simulink model "QuarterCarSuspension_JAM"  (R2024b)
settings: Solver=ode45  StartTime=0.0  StopTime=10  MaxStep=0.01  RelTol=1e-3  AbsTol=1e-6
StopFcn:
  | if exist('sldemo_suspn_output')
  | sldemo_suspgraph
  | end
model workspace (MATLAB code in the model file):
  | sldemo_suspdat; %load data from file
values from neighbouring files (symbols this model uses):
  cs = 2500    [QuarterCar_dat.m]
  ks = 28000    [QuarterCar_dat.m]
  kt = 190000    [QuarterCar_dat.m]
  Mb = 300    [QuarterCar_dat.m]
  Mu = 40    [QuarterCar_dat.m]
CloseFcn:
  | if exist('suspnFigH')
  |   if ishghandle(suspnFigH,'figure')
  |     close(suspnFigH)
  |   end
  |   clear suspnFigH
  | end
  | if exist('suspnAxH'), clear suspnAxH; end
Description:
  | Automotive Suspension
  | 
  | This example shows how to model a simplified half-car model that includes an independent
  | front and rear vertical suspension. The model also includes body pitch and
  | bounce degrees of freedom. The example provides a description of the model to
  | show how simulation can be used for investigating ride characteristics.
  | In conjunction with a powertrain simulation, the model could
  | investigate longitudinal shuffle resulting from changes in throttle setting.
settings Model: ModifiedByFormat=The MathWorks, Inc.  Creator=The MathWorks, Inc.  LastModifiedBy=The MathWorks, Inc.
settings SolverCC: AutoScaleAbsTol=off  AlgebraicLoopSolver=TrustRegion  MaxZcPerStep=1
settings DataIOCC: InitialState=x0  SaveFormat=StructureWithTime  SaveOutput=off  SaveTime=off  ReturnWorkspaceOutputs=off  StateSaveName=x  TimeSaveName=t  SignalLoggingName=sldemo_suspn_output
settings OptimizationCC: ReuseModelBlockBuffer=off  ExpressionDepthLimit=2147483647  InitFltsAndDblsToZero=on  LifeSpan=inf  BufferReusableBoundary=off
settings DebuggingCC: SaveWithParameterizedLinksMsg=none  SignalResolutionControl=TryResolveAllWithWarning  MultiTaskDSMMsg=warning  SigSpecEnsureSampleTimeMsg=none  IntegerOverflowMsg=none  FcnCallInpInsideContextMsg=warning  UnconnectedInputMsg=warning  UnconnectedOutputMsg=warning  UnconnectedLineMsg=warning  BusObjectLabelMismatch=none  StateNameClashWarn=warning  SFUnexpectedBacktrackingDiag=warning  SFNoUnconditionalDefaultTransitionDiag=warning  SFExecutionAtInitializationDiag=none  IntegerSaturationMsg=none  ArithmeticOperatorsInVariantConditions=warning
settings HardwareCC: ProdBitPerPointer=32  ProdBitPerSizeT=32  ProdBitPerPtrDiffT=32  ProdLargestAtomicFloat=None  ProdIntDivRoundTo=Undefined  ProdEndianess=Unspecified  ProdWordSize=32  ProdHWDeviceType=32-bit Generic
settings ModelReferenceCC: EnableRefExpFcnMdlSchedulingChecks=on  PropagateSignalLabelsOutOfModel=off
settings SFSimCC: SimUseLocalCustomCode=off  CustomCodeUndefinedFunction=UseInterfaceOnly
settings RTWCC: RTWUseLocalCustomCode=off  GPUComputeCapability=3.5  DLArmComputeVersion=19.05
settings CodeAppCC: StateflowObjectComments=on
settings GRTTargetCC: TargetFcnLib=ansi_tfl_tmw.mat  TargetLangStandard=C89/C90 (ANSI)  CombineOutputUpdateFcns=off  GRTInterface=on
settings ConfigComp: CovMetricSettings=dw  CovSaveCumulativeToWorkspaceVar=on  CovSaveSingleToWorkspaceVar=on  CovExternalEMLEnable=off  CovSFcnEnable=off

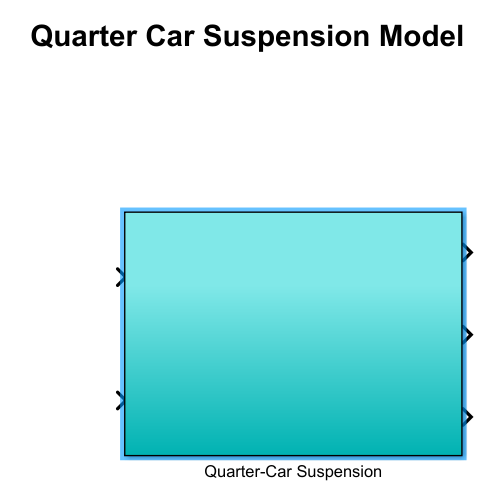
[thumbnail: Simulink's stored preview of the top-level diagram]
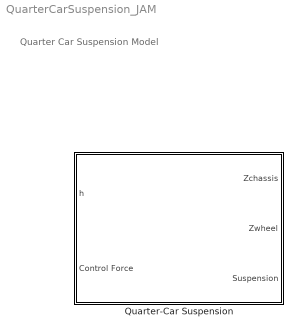
== system QuarterCarSuspension_JAM ==
  note: Quarter Car Suspension Model
  Quarter-Car Suspension : Subsystem

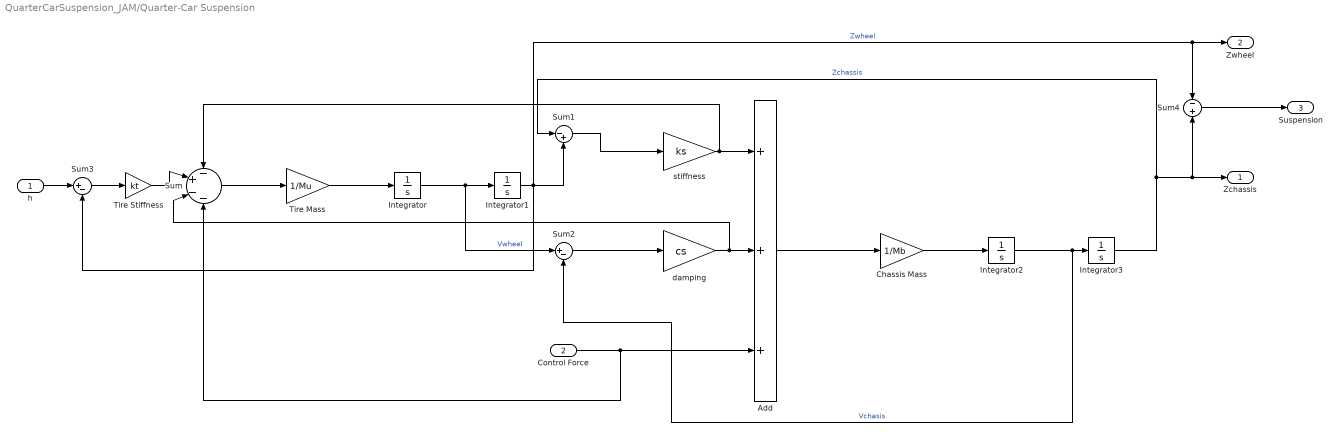
== system QuarterCarSuspension_JAM/Quarter-Car Suspension ==
  h : Inport
  Control Force : Inport  Port=2
  Add : Sum  Inputs=+++
  Chassis Mass : Gain  Gain=1/Mb
  Integrator{,1..3} (4 alike) : Integrator
  Sum : Sum  Inputs=-+--
  Sum1 : Sum  Inputs=|-+
  Sum2 : Sum  Inputs=|+-
  Sum3 : Sum  Inputs=|+-
  Sum4 : Sum  Inputs=-+
  Tire Mass : Gain  Gain=1/Mu
  Tire Stiffness : Gain  Gain=kt
  damping : Gain  Gain=cs  SaturateOnIntegerOverflow=on  OutDataTypeStr=Inherit: Same as input  ParamDataTypeStr=Inherit: Same as input
  stiffness : Gain  Gain=ks  SaturateOnIntegerOverflow=on  OutDataTypeStr=Inherit: Same as input  ParamDataTypeStr=Inherit: Same as input
  Zchassis : Outport
  Zwheel : Outport  Port=2
  Suspension : Outport  Port=3
  wires:
  Tire Stiffness/1 -> Sum/2
  Tire Mass/1 -> Integrator/1
  Integrator/1 -> Sum2/1, Integrator1/1  "Vwheel"
  Integrator1/1 -> Sum3/2, Sum4/1, Zwheel/1, Sum1/2  "Zwheel"
  Sum1/1 -> stiffness/1
  Sum2/1 -> damping/1
  damping/1 -> Sum/3, Add/2
  stiffness/1 -> Sum/1, Add/1
  Control Force/1 -> Add/3, Sum/4
  Sum/1 -> Tire Mass/1
  Chassis Mass/1 -> Integrator2/1
  Integrator3/1 -> Sum4/2, Zchassis/1, Sum1/1  "Zchassis"
  Integrator2/1 -> Sum2/2, Integrator3/1  "Vchasis"
  Add/1 -> Chassis Mass/1
  h/1 -> Sum3/1
  Sum3/1 -> Tire Stiffness/1
  Sum4/1 -> Suspension/1
